simulink model "copia"  (R2019a)
settings: Solver=VariableStepAuto  StartTime=0.0  StopTime=1005  RelTol=1e-3
values from neighbouring files (symbols this model uses):
  alfa_cu = 3.9 * 10^(-3)    (= 0.0039)    [Datos.m]
  ba = 0.0113    [Calculo.m]
  beq = (bm+bl/r^2)    [Calculo.m]    (also in Untitled4.m; funciontrans.m)
  bm = 1.5 * 10^(-5)    (= 1.5e-05)    [Datos.m]
  Cts = 0.818    [Datos.m]
  Id0 = 0.5    [Datos.m]    (also in punto6plot.m)
  Jeq = (Jm+Jl/r^2)    [Calculo.m]    (also in Untitled4.m)
  Jeq1 = (Jm+Jlv(i)/r^2)    [Calculo.m]    (also in funciontrans.m)
  Koth = 6400    [Calculo.m]
  Kow = 3200^2    (= 10240000)    [Calculo.m]
  ksa = 9.04    [Calculo.m]
  ksia = 2892.8    [Calculo.m]
  lambda_m_r = 0.01546    [Datos.m]
  Ld = 6.6e-3    (= 0.0066)    [Datos.m]
  Lls = 0.8e-3    (= 0.0008)    [Datos.m]
  Lq = 5.8e-3    (= 0.0058)    [Datos.m]
  Pp = 3    [Datos.m]
  r = 314.3008    [Datos.m]
  Rts_amb = 146.7    [Datos.m]
undefined symbols (not defined in the file or in its folder): KowI, KT, KTd, magnitude, R0, Rd, Rq, sigbuilder_block, Tau, W0, W1
settings Model: Creator=renzo  LastModifiedBy=renzo

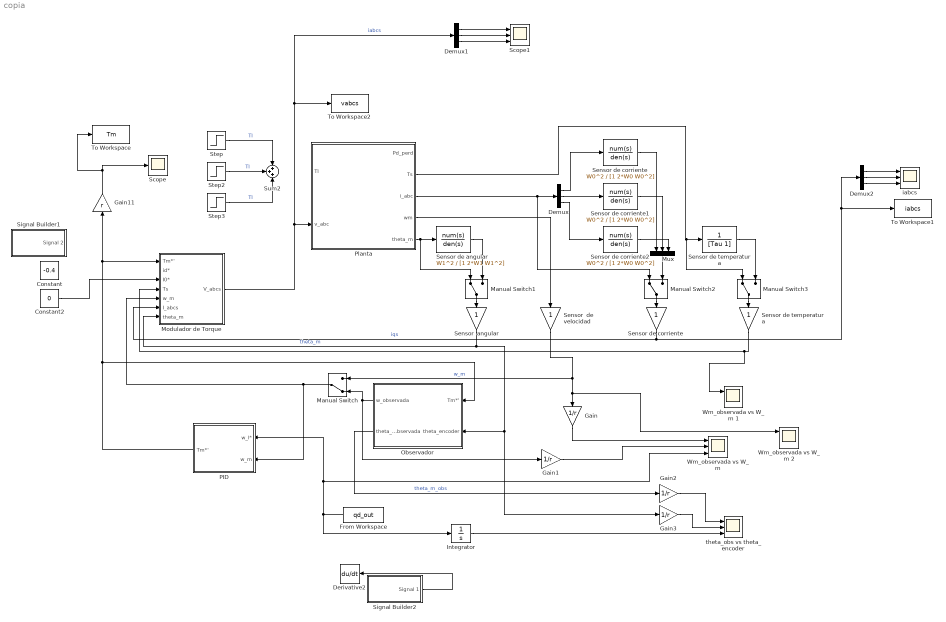
== system copia ==
  Constant : Constant  Value=-0.4
  Constant2 : Constant  Value=0
  Demux : Demux  Outputs=3
  Demux1 : Demux  Outputs=3
  Demux2 : Demux  Outputs=3
  Derivative2 : Derivative
  From Workspace : FromWorkspace  VariableName=qd_out  SampleTime=0
  Gain{,1..3} (4 alike) : Gain  Gain=1/r
  Gain11 : Gain  Gain=r
  Integrator : Integrator
  Manual Switch : ManualSwitch  CurrentSetting=0
  Manual Switch1 : ManualSwitch
  Manual Switch2 : ManualSwitch
  Manual Switch3 : ManualSwitch
  Modulador de Torque : Subsystem
  Mux : Mux  Inputs=3
  Observador : Subsystem
  PID : Subsystem
  Planta : Subsystem
  Scope : Scope
  Scope1 : Scope  NumInputPorts=3
  Sensor  angular : Gain
  Sensor  de velocidad : Gain
  Sensor de angular : TransferFcn  Numerator=W1^2  Denominator=[1 2*W1 W1^2]
  Sensor de corriente : TransferFcn  Numerator=W0^2  Denominator=[1 2*W0 W0^2]
  "Sensor de corriente " : Gain
  Sensor de corriente1 : TransferFcn  Numerator=W0^2  Denominator=[1 2*W0 W0^2]
  Sensor de corriente2 : TransferFcn  Numerator=W0^2  Denominator=[1 2*W0 W0^2]
  Sensor de temperatura : TransferFcn  Numerator=1  Denominator=[Tau 1]
  "Sensor de temperatura " : Gain
  Signal Builder1 : Subsystem  Tag=STV Subsys  LoadFcn=sigbuilder_block('load');  StartFcn=sigbuilder_block('start');  StopFcn=sigbuilder_block('stop');  ClipboardFcn=sigbuilder_block('clipboard');  mask(Sigbuilder block){tuvar=[0:10]}
      mask help: Simulink:masks:SigbuilderBlock_MD
      mask init:
      | if ~strcmp(get_param(bdroot(gcbh),'SimulationStatus'),'stopped') tuvar = sigbuilder_block('maskInit'); end
      settings: CopyFcn=sigbuilder_block('copy');  DeleteFcn=sigbuilder_block('delete');  ModelCloseFcn=sigbuilder_block('modelClose');  PreSaveFcn=sigbuilder_block('preSave');  PauseFcn=sigbuilder_block('pause');  ContinueFcn=sigbuilder_block('continue');  NameChangeFcn=sigbuilder_block('namechange');  OpenFcn=sigbuilder_block('open',[6 126.75 550.5 359.25 ]);  CloseFcn=sigbuilder_block('close');
      mask Display: plot(0, 0, 100, 100,[2, 2, 32, 32, 2], [68, 8, 8, 68, 68],[32, 2], [38, 38], [32, 19, 2],[53, 60, 44], [32, 17, 17, 2],[16, 16, 31, 31]);txt = getActiveGroup(gcbh);text(2, 100, txt,'verticalAlignment', 'top');
  Signal Builder2 : Subsystem  Tag=STV Subsys  LoadFcn=sigbuilder_block('load');  StartFcn=sigbuilder_block('start');  StopFcn=sigbuilder_block('stop');  ClipboardFcn=sigbuilder_block('clipboard');  mask(Sigbuilder block){tuvar=[0:10]}
      mask help: Simulink:masks:SigbuilderBlock_MD
      mask init:
      | if ~strcmp(get_param(bdroot(gcbh),'SimulationStatus'),'stopped') tuvar = sigbuilder_block('maskInit'); end
      settings: CopyFcn=sigbuilder_block('copy');  DeleteFcn=sigbuilder_block('delete');  ModelCloseFcn=sigbuilder_block('modelClose');  PreSaveFcn=sigbuilder_block('preSave');  PauseFcn=sigbuilder_block('pause');  ContinueFcn=sigbuilder_block('continue');  NameChangeFcn=sigbuilder_block('namechange');  OpenFcn=sigbuilder_block('open',[437.6 153 550.4 359.25 ]);  CloseFcn=sigbuilder_block('close');
      mask Display: plot(0, 0, 100, 100,[2, 2, 32, 32, 2], [68, 8, 8, 68, 68],[32, 2], [38, 38], [32, 19, 2],[53, 60, 44], [32, 17, 17, 2],[16, 16, 31, 31]);txt = getActiveGroup(gcbh);text(2, 100, txt,'verticalAlignment', 'top');
  Step : Step  Time=0.3  After=6.28  SampleTime=0
  Step2 : Step  Time=0.5  After=-2*6.28  SampleTime=0
  Step3 : Step  Time=0.9  After=6.28  SampleTime=0
  Sum2 : Sum  Inputs=+++
  To Workspace : ToWorkspace  VariableName=Tm  SaveFormat=Timeseries  SampleTime=-1
  To Workspace1 : ToWorkspace  VariableName=iabcs  SaveFormat=Timeseries  SampleTime=-1
  To Workspace2 : ToWorkspace  VariableName=vabcs  SaveFormat=Timeseries  SampleTime=-1
  "Wm_observada vs W_m " : Scope  NumInputPorts=3
  Wm_observada vs W_m 1 : Scope  NumInputPorts=3
  Wm_observada vs W_m 2 : Scope  NumInputPorts=3
  iabcs : Scope  NumInputPorts=3
  theta_obs vs theta_encoder : Scope  NumInputPorts=3
  wires:
  Planta/3(i_abc) -> Manual Switch2/1, Demux/1
  Planta/4(wm) -> Sensor  de velocidad/1
  Sensor  angular/1 -> Observador/2(theta_encoder), Gain3/1, Modulador de Torque/7(theta_m)  "theta_m"
  Manual Switch/1 -> PID/2(w_m), Modulador de Torque/5("w_m ")
  "Sensor de corriente "/1 -> To Workspace1/1, Demux2/1, Modulador de Torque/6(I_abcs)  "iqs"
  "Sensor de temperatura "/1 -> Wm_observada vs W_m 1/1, Modulador de Torque/4(Ts)
  Gain/1 -> "Wm_observada vs W_m "/1
  Observador/2(theta_observada) -> Gain2/1  "theta_m_obs"
  Gain1/1 -> "Wm_observada vs W_m "/2
  Gain2/1 -> theta_obs vs theta_encoder/1
  Gain3/1 -> theta_obs vs theta_encoder/2
  Sensor  de velocidad/1 -> Manual Switch/1, Wm_observada vs W_m 2/1, Gain/1  "w_m"
  Observador/1(w_observada) -> Gain1/1, Manual Switch/2
  Step2/1 -> Sum2/2  "Tl"
  Step/1 -> Sum2/1  "Tl"
  Step3/1 -> Sum2/3  "Tl"
  Constant2/1 -> Modulador de Torque/3(I0*)
  PID/1(Tm*') -> Observador/1(Tm*'), Gain11/1, Modulador de Torque/1(Tm*')
  Demux/1 -> Sensor de corriente/1
  Demux/2 -> Sensor de corriente1/1
  Demux/3 -> Sensor de corriente2/1
  Mux/1 -> Manual Switch2/2
  Sensor de corriente/1 -> Mux/1
  Sensor de corriente1/1 -> Mux/2
  Sensor de corriente2/1 -> Mux/3
  Planta/2(Ts) -> Manual Switch3/1, Sensor de temperatura/1
  Planta/5(theta_m) -> Sensor de angular/1, Manual Switch1/1
  Sensor de angular/1 -> Manual Switch1/2
  Integrator/1 -> theta_obs vs theta_encoder/3
  Manual Switch1/1 -> Sensor  angular/1
  Manual Switch3/1 -> "Sensor de temperatura "/1
  Sensor de temperatura/1 -> Manual Switch3/2
  Manual Switch2/1 -> "Sensor de corriente "/1
  Gain11/1 -> To Workspace/1, Scope/1
  Signal Builder2/1(Signal 1) -> Derivative2/1
  Modulador de Torque/1(V_abcs) -> Demux1/1, To Workspace2/1, Planta/2(v_abc)  "iabcs"
  Demux1/2 -> Scope1/2
  Demux1/1 -> Scope1/1
  Demux1/3 -> Scope1/3
  Demux2/1 -> iabcs/1
  Demux2/2 -> iabcs/2
  Demux2/3 -> iabcs/3
  From Workspace/1 -> Integrator/1, "Wm_observada vs W_m "/3, PID/1(w_l*)

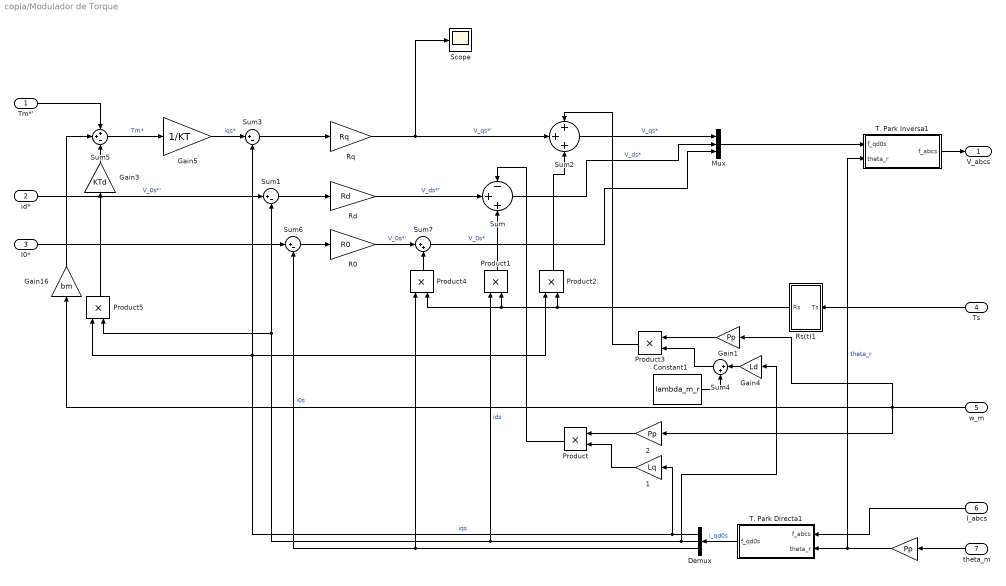
== system copia/Modulador de Torque ==
  Tm*' : Inport
  id* : Inport  Port=2
  I0* : Inport  Port=3
  Ts : Inport  Port=4
  "w_m " : Inport  Port=5
  I_abcs : Inport  Port=6
  theta_m : Inport  Port=7
  " " : Gain  Gain=Pp
  " 1" : Gain  Gain=Lq
  " 2" : Gain  Gain=Pp
  Constant1 : Constant  Value=lambda_m_r
  Demux : Demux  Outputs=3
  Gain1 : Gain  Gain=Pp
  Gain16 : Gain  Gain=bm
  Gain3 : Gain  Gain=KTd
  Gain4 : Gain  Gain=Ld
  Gain5 : Gain  Gain=1/KT
  Mux : Mux  Inputs=3
  Product{,1..5} (6 alike) : Product
  R0 : Gain  Gain=R0
  Rd : Gain  Gain=Rd
  Rq : Gain  Gain=Rq
  Rs(t)1 : Subsystem
  Scope : Scope
  Sum : Sum  Inputs=-++
  Sum1 : Sum  Inputs=|+-
  Sum2 : Sum  Inputs=+++
  Sum3 : Sum  Inputs=|+-
  Sum4 : Sum  Inputs=|++
  Sum5 : Sum  Inputs=++-
  Sum6 : Sum  Inputs=|+-
  Sum7 : Sum  Inputs=|++
  T. Park Directa1 : Subsystem
  T. Park Inversa1 : Subsystem
  V_abcs : Outport
  wires:
  theta_m/1 -> " "/1
  Product3/1 -> Sum2/1
  Rs(t)1/1(Rs) -> Product2/2, Product1/2, Product4/2
  Sum/1 -> Mux/2  "V_ds*"
  Product1/1 -> Sum/3
  Sum1/1 -> Rd/1
  Demux/3 -> Sum6/2, Product4/1  "i0s"
  Rd/1 -> Sum/2  "V_ds*'"
  Gain16/1 -> Sum5/2
  Sum2/1 -> Mux/1  "V_qs*"
  Gain4/1 -> Sum4/1
  Sum6/1 -> R0/1
  Sum4/1 -> Product3/2
  Product2/1 -> Sum2/3
  " "/1 -> T. Park Directa1/2(theta_r), T. Park Inversa1/2(theta_r)  "theta_r"
  Sum7/1 -> Mux/3  "V_0s*"
  Mux/1 -> T. Park Inversa1/1(f_qd0s)
  T. Park Directa1/1(f_qd0s) -> Demux/1  "i_qd0s"
  Product/1 -> Sum/1
  Tm*'/1 -> Sum5/1
  Sum5/1 -> Gain5/1  "Tm*"
  " 1"/1 -> Product/2
  Demux/1 -> " 1"/1, Product2/1, Product5/1, Sum3/2  "iqs"
  Sum3/1 -> Rq/1
  I0*/1 -> Sum6/1
  Demux/2 -> Gain4/1, Product5/2, Sum1/2, Product1/1  "ids"
  Rq/1 -> Scope/1, Sum2/2  "V_qs*'"
  Constant1/1 -> Sum4/2
  T. Park Inversa1/1(f_abcs) -> V_abcs/1
  R0/1 -> Sum7/1  "V_0s*'"
  " 2"/1 -> Product/1
  I_abcs/1 -> T. Park Directa1/1(f_abcs)
  Product4/1 -> Sum7/2
  Gain1/1 -> Product3/1
  Ts/1 -> Rs(t)1/1(Ts)
  "w_m "/1 -> " 2"/1, Gain16/1, Gain1/1
  Gain5/1 -> Sum3/1  "iqs*"
  Product5/1 -> Gain3/1
  Gain3/1 -> Sum5/3
  id*/1 -> Sum1/1  "V_0s*'"

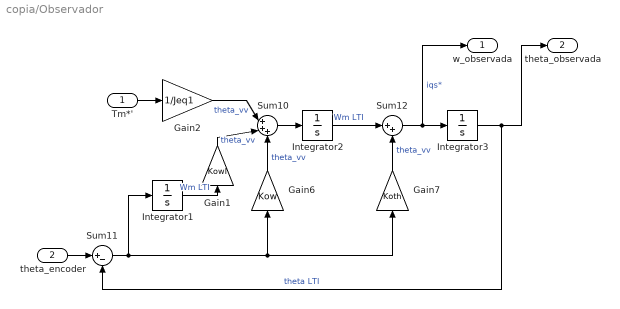
== system copia/Observador ==
  Tm*' : Inport
  theta_encoder : Inport  Port=2
  Gain1 : Gain  Gain=KowI
  Gain2 : Gain  Gain=1/Jeq1
  Gain6 : Gain  Gain=Kow
  Gain7 : Gain  Gain=Koth
  Integrator1 : Integrator
  Integrator2 : Integrator
  Integrator3 : Integrator
  Sum10 : Sum  Inputs=|+++
  Sum11 : Sum  Inputs=|+-
  Sum12 : Sum  Inputs=|++
  w_observada : Outport
  theta_observada : Outport  Port=2
  wires:
  Gain6/1 -> Sum10/3  "theta_vv"
  Sum10/1 -> Integrator2/1
  Gain2/1 -> Sum10/1  "theta_vv"
  Integrator2/1 -> Sum12/1  "Wm LTI"
  Gain7/1 -> Sum12/2  "theta_vv"
  Sum12/1 -> w_observada/1, Integrator3/1  "iqs*"
  Integrator3/1 -> theta_observada/1, Sum11/2  "theta LTI"
  Tm*'/1 -> Gain2/1
  theta_encoder/1 -> Sum11/1
  Sum11/1 -> Integrator1/1, Gain7/1, Gain6/1
  Integrator1/1 -> Gain1/1  "Wm LTI"
  Gain1/1 -> Sum10/2  "theta_vv"

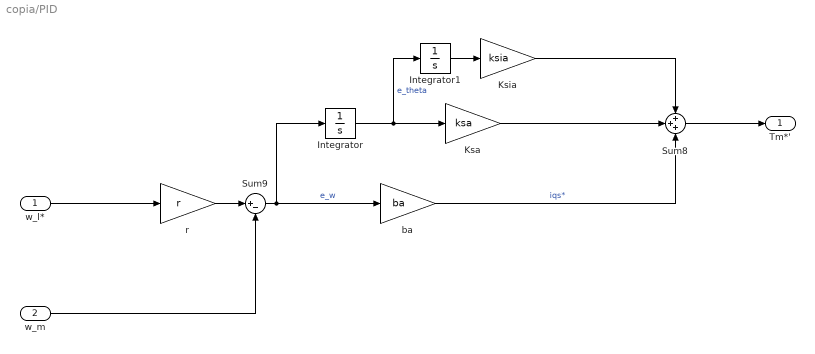
== system copia/PID ==
  w_l* : Inport
  w_m : Inport  Port=2
  Integrator : Integrator
  Integrator1 : Integrator
  Ksa : Gain  Gain=ksa
  Ksia : Gain  Gain=ksia
  Sum8 : Sum  Inputs=+++
  Sum9 : Sum  Inputs=|+-
  ba : Gain  Gain=ba
  r : Gain  Gain=r
  Tm*' : Outport
  wires:
  Integrator/1 -> Integrator1/1, Ksa/1  "e_theta"
  Sum9/1 -> Integrator/1, ba/1  "e_w"
  Ksa/1 -> Sum8/2
  ba/1 -> Sum8/3  "iqs*"
  Ksia/1 -> Sum8/1
  r/1 -> Sum9/1
  w_m/1 -> Sum9/2
  Integrator1/1 -> Ksia/1
  w_l*/1 -> r/1
  Sum8/1 -> Tm*'/1

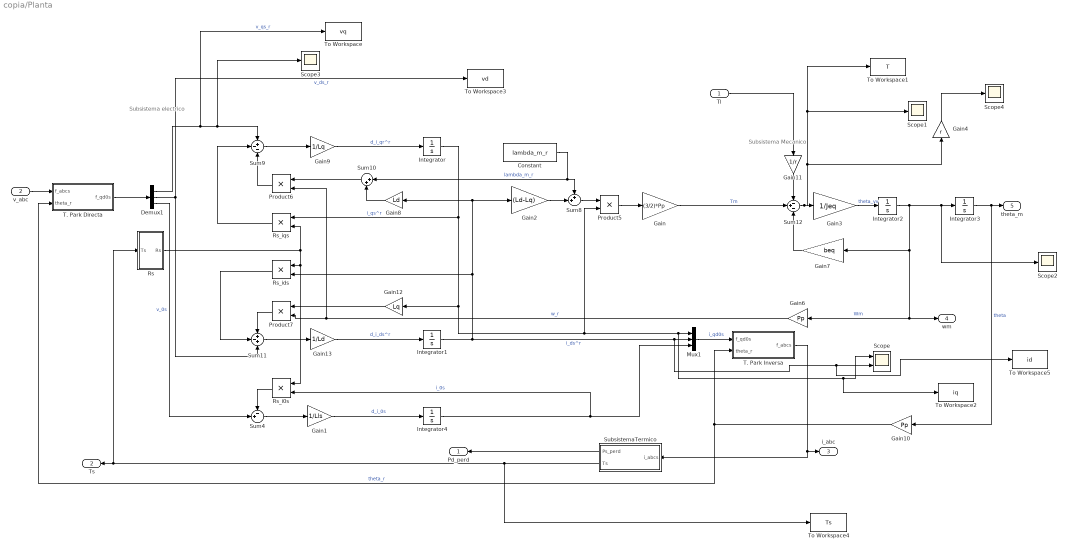
== system copia/Planta ==
  note: Subsistema Mecanico
  note: Subsistema electrico
  Tl : Inport
  v_abc : Inport  Port=2
  Constant : Constant  Value=lambda_m_r
  Demux1 : Demux  Outputs=3
  Gain : Gain  Gain=(3/2)*Pp
  Gain1 : Gain  Gain=1/Lls
  Gain10 : Gain  Gain=Pp
  Gain11 : Gain  Gain=1/r
  Gain12 : Gain  Gain=Lq
  Gain13 : Gain  Gain=1/Ld
  Gain2 : Gain  Gain=(Ld-Lq)
  Gain3 : Gain  Gain=1/Jeq
  Gain4 : Gain  Gain=r
  Gain6 : Gain  Gain=Pp
  Gain7 : Gain  Gain=beq
  Gain8 : Gain  Gain=Ld
  Gain9 : Gain  Gain=1/Lq
  Integrator{,2..4} (4 alike) : Integrator
  Integrator1 : Integrator  InitialCondition=Id0
  Mux1 : Mux  Inputs=3
  Product5 : Product
  Product6 : Product
  Product7 : Product
  Rs : Subsystem
  Rs_i0s : Product
  Rs_ids : Product
  Rs_iqs : Product
  Scope : Scope  NumInputPorts=2
  Scope{1..4} (4 alike) : Scope
  SubsistemaTermico : Subsystem
  Sum10 : Sum  Inputs=|++
  Sum11 : Sum  Inputs=+-+
  Sum12 : Sum  Inputs=-+-
  Sum4 : Sum  Inputs=-+|
  Sum8 : Sum  Inputs=++|
  Sum9 : Sum  Inputs=+--
  T. Park Directa : Subsystem
  T. Park Inversa : Subsystem
  To Workspace : ToWorkspace  VariableName=vq  SaveFormat=Timeseries  SampleTime=-1
  To Workspace1 : ToWorkspace  VariableName=T  SaveFormat=Timeseries  SampleTime=-1
  To Workspace2 : ToWorkspace  VariableName=iq  SaveFormat=Timeseries  SampleTime=-1
  To Workspace3 : ToWorkspace  VariableName=vd  SaveFormat=Timeseries  SampleTime=-1
  To Workspace4 : ToWorkspace  VariableName=Ts  SaveFormat=Timeseries  SampleTime=-1
  To Workspace5 : ToWorkspace  VariableName=id  SaveFormat=Timeseries  SampleTime=-1
  Pd_perd : Outport
  Ts : Outport  Port=2
  i_abc : Outport  Port=3
  wm : Outport  Port=4
  theta_m : Outport  Port=5
  wires:
  T. Park Inversa/1(f_abcs) -> SubsistemaTermico/1(i_abcs), i_abc/1
  SubsistemaTermico/1(Ps_perd) -> Pd_perd/1
  Gain10/1 -> T. Park Directa/2(theta_r), T. Park Inversa/2(theta_r)  "theta_r"
  Mux1/1 -> T. Park Inversa/1(f_qd0s)  "i_qd0s"
  v_abc/1 -> T. Park Directa/1(f_abcs)
  Gain6/1 -> Product6/2, Product7/2  "w_r"
  Sum8/1 -> Product5/1
  T. Park Directa/1(f_qd0s) -> Demux1/1
  Gain9/1 -> Integrator/1  "d_i_qr^r"
  Gain12/1 -> Product7/1
  Demux1/2 -> Sum11/3, To Workspace3/1  "v_ds_r"
  Rs_i0s/1 -> Sum4/1
  Rs_ids/1 -> Sum11/2
  Demux1/3 -> Sum4/2  "v_0s"
  Gain8/1 -> Sum10/2
  Sum4/1 -> Gain1/1
  Sum10/1 -> Product6/1
  Gain2/1 -> Sum8/2
  Product7/1 -> Sum11/1
  Rs_iqs/1 -> Sum9/2
  Sum11/1 -> Gain13/1
  SubsistemaTermico/2(Ts) -> To Workspace4/1, Rs/1(Ts), Ts/1
  Gain1/1 -> Integrator4/1  "d_i_0s"
  Integrator4/1 -> Mux1/3, Rs_i0s/2  "i_0s"
  Rs/1(Rs) -> Rs_i0s/1, Rs_ids/1, Rs_iqs/2
  Sum9/1 -> Gain9/1
  Integrator1/1 -> To Workspace5/1, Scope/2, Mux1/2, Rs_ids/2, Gain2/1, Gain8/1  "i_ds^r"
  Product6/1 -> Sum9/3
  Integrator/1 -> Gain12/1, To Workspace2/1, Scope/1, Mux1/1, Product5/2, Rs_iqs/1  "i_qs^r"
  Constant/1 -> Sum8/1, Sum10/1  "lambda_m_r"
  Demux1/1 -> To Workspace/1, Scope3/1, Sum9/1  "v_qs_r"
  Gain13/1 -> Integrator1/1  "d_i_ds^r"
  Tl/1 -> Gain11/1
  Integrator3/1 -> Gain10/1, theta_m/1  "theta"
  Gain11/1 -> Sum12/1
  Integrator2/1 -> Scope2/1, Integrator3/1, Gain7/1, Gain6/1, wm/1  "Wm"
  Product5/1 -> Gain/1
  Gain/1 -> Sum12/2  "Tm"
  Gain3/1 -> Integrator2/1  "theta_vv"
  Gain7/1 -> Sum12/3
  Sum12/1 -> Gain4/1, Scope1/1, To Workspace1/1, Gain3/1
  Gain4/1 -> Scope4/1

== system copia/Signal Builder1 ==
  Demux : Demux  Tag=STV Demux  Outputs=1
  FromWs : FromWorkspace  Tag=STV FromWs  VariableName=tuvar  SampleTime=0
      SigBuilderData=|
      | common.afterFinalStr = 'Extrapolate'
      | common.sampleTime = 0
      | dataSet.timeRange = [0 10]
      | dataSet.name = 'Group 1'
      | sbobj.Groups.Name = 'Group 1'
      | sbobj.Groups.Signals.Name = 'Signal 2'
      | sbobj.Groups.Signals.XData = [0 0.1 0.1 0.7 0.7 10]
      | sbobj.Groups.Signals.YData = [0 0 0.0063 0.0063 0 0]
  Signal 2 : Outport  Tag=STV Outport
  wires:
  FromWs/1 -> Demux/1
  Demux/1 -> Signal 2/1

== system copia/Signal Builder2 ==
  Demux : Demux  Tag=STV Demux  Outputs=1
  FromWs : FromWorkspace  Tag=STV FromWs  VariableName=tuvar  SampleTime=0
      SigBuilderData=|
      | common.afterFinalStr = 'Extrapolate'
      | common.sampleTime = 0
      | dataSet.timeRange = [0 20]
      | dataSet.name = 'Group 1'
      | sbobj.Groups.Name = 'Group 1'
      | sbobj.Groups.Signals.Name = 'Signal 1'
      | sbobj.Groups.Signals.XData = [0 1 6 11 16 20]
      | sbobj.Groups.Signals.YData = [0 0 6.28318530718 6.28318530718 0 0]
      | sbobj.Groups.TimeRange = [0 20]
  Signal 1 : Outport  Tag=STV Outport
  wires:
  Demux/1 -> Signal 1/1
  FromWs/1 -> Demux/1

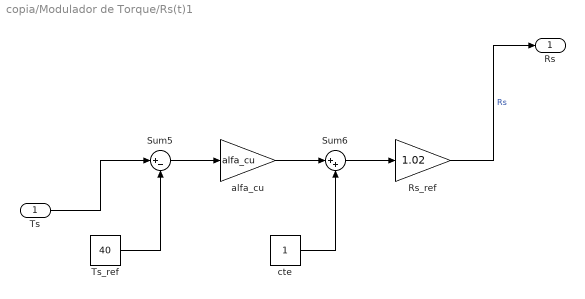
== system copia/Modulador de Torque/Rs(t)1 ==
  Ts : Inport
  Rs_ref : Gain  Gain=1.02
  Sum5 : Sum  Inputs=|+-
  Sum6 : Sum  Inputs=|++
  Ts_ref : Constant  Value=40
  alfa_cu : Gain  Gain=alfa_cu
  cte : Constant
  Rs : Outport
  wires:
  alfa_cu/1 -> Sum6/1
  Sum6/1 -> Rs_ref/1
  Rs_ref/1 -> Rs/1  "Rs"
  Ts_ref/1 -> Sum5/2
  cte/1 -> Sum6/2
  Ts/1 -> Sum5/1
  Sum5/1 -> alfa_cu/1

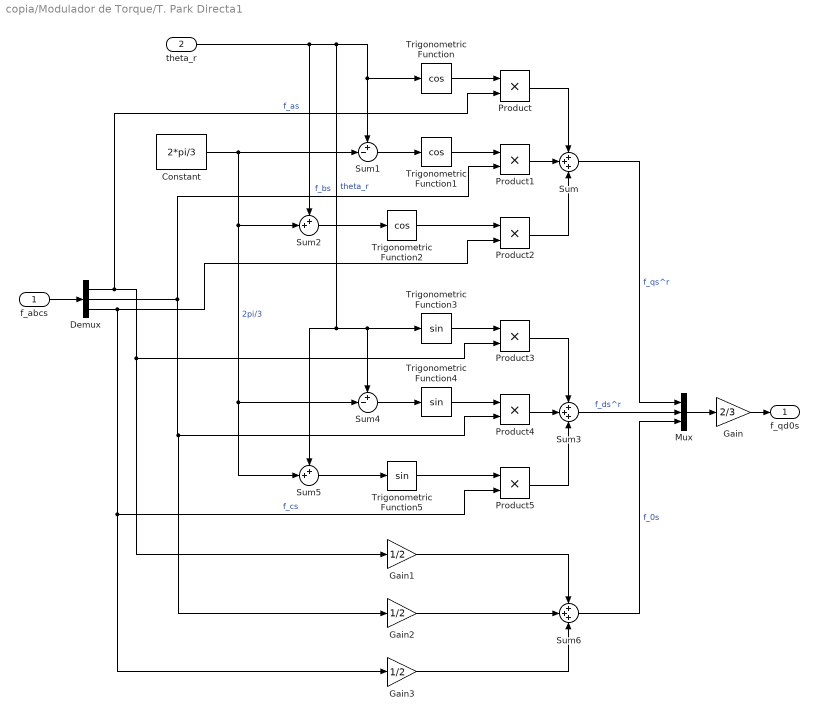
== system copia/Modulador de Torque/T. Park Directa1 ==
  f_abcs : Inport
  theta_r : Inport  Port=2
  Constant : Constant  Value=2*pi/3
  Demux : Demux  Outputs=3
  Gain : Gain  Gain=2/3
  Gain1 : Gain  Gain=1/2
  Gain2 : Gain  Gain=1/2
  Gain3 : Gain  Gain=1/2
  Mux : Mux  Inputs=3
  Product{,1..5} (6 alike) : Product
  Sum : Sum  Inputs=3
  Sum1 : Sum  Inputs=+-|
  Sum2 : Sum  Inputs=++|
  Sum3 : Sum  Inputs=3
  Sum4 : Sum  Inputs=+-|
  Sum5 : Sum  Inputs=++|
  Sum6 : Sum  Inputs=3
  Trigonometric Function : Trigonometry  Operator=cos
  Trigonometric Function1 : Trigonometry  Operator=cos
  Trigonometric Function2 : Trigonometry  Operator=cos
  Trigonometric Function3 : Trigonometry
  Trigonometric Function4 : Trigonometry
  Trigonometric Function5 : Trigonometry
  f_qd0s : Outport  VectorParamsAs1DForOutWhenUnconnected=on
  wires:
  Mux/1 -> Gain/1
  f_abcs/1 -> Demux/1
  Demux/1 -> Gain1/1, Product3/2, Product/2  "f_as"
  Demux/2 -> Gain2/1, Product4/2, Product1/2  "f_bs"
  Demux/3 -> Gain3/1, Product5/2, Product2/2  "f_cs"
  Sum/1 -> Mux/1  "f_qs^r"
  Gain/1 -> f_qd0s/1
  Trigonometric Function/1 -> Product/1
  Product/1 -> Sum/1
  Sum1/1 -> Trigonometric Function1/1
  Constant/1 -> Sum5/2, Sum4/2, Sum2/2, Sum1/2  "2pi/3"
  Trigonometric Function1/1 -> Product1/1
  Product1/1 -> Sum/2
  Product2/1 -> Sum/3
  Trigonometric Function2/1 -> Product2/1
  Sum2/1 -> Trigonometric Function2/1
  Product4/1 -> Sum3/2
  Trigonometric Function5/1 -> Product5/1
  Sum5/1 -> Trigonometric Function5/1
  Product5/1 -> Sum3/3
  Product3/1 -> Sum3/1
  Trigonometric Function4/1 -> Product4/1
  Sum4/1 -> Trigonometric Function4/1
  Sum3/1 -> Mux/2  "f_ds^r"
  Trigonometric Function3/1 -> Product3/1
  theta_r/1 -> Sum5/1, Sum4/1, Trigonometric Function3/1, Trigonometric Function/1, Sum1/1, Sum2/1  "theta_r"
  Sum6/1 -> Mux/3  "f_0s"
  Gain3/1 -> Sum6/3
  Gain1/1 -> Sum6/1
  Gain2/1 -> Sum6/2

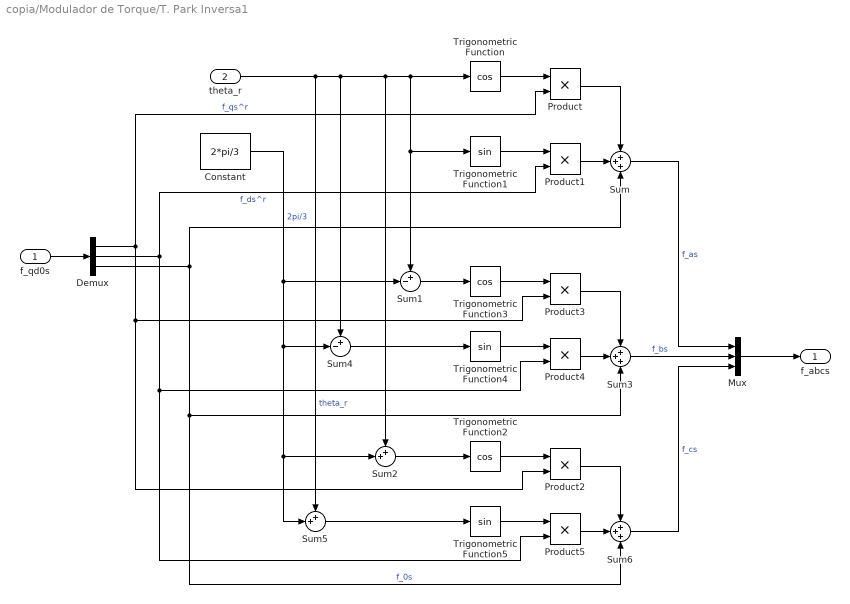
== system copia/Modulador de Torque/T. Park Inversa1 ==
  f_qd0s : Inport
  theta_r : Inport  Port=2
  Constant : Constant  Value=2*pi/3
  Demux : Demux  Outputs=3
  Mux : Mux  Inputs=3
  Product{,1..5} (6 alike) : Product
  Sum : Sum  Inputs=3
  Sum1 : Sum  Inputs=+-|
  Sum2 : Sum  Inputs=++|
  Sum3 : Sum  Inputs=3
  Sum4 : Sum  Inputs=+-|
  Sum5 : Sum  Inputs=++|
  Sum6 : Sum  Inputs=3
  Trigonometric Function : Trigonometry  Operator=cos
  Trigonometric Function1 : Trigonometry
  Trigonometric Function2 : Trigonometry  Operator=cos
  Trigonometric Function3 : Trigonometry  Operator=cos
  Trigonometric Function4 : Trigonometry
  Trigonometric Function5 : Trigonometry
  f_abcs : Outport  VectorParamsAs1DForOutWhenUnconnected=on
  wires:
  Trigonometric Function4/1 -> Product4/1
  f_qd0s/1 -> Demux/1
  Trigonometric Function/1 -> Product/1
  Constant/1 -> Sum1/2, Sum4/2, Sum2/2, Sum5/2  "2pi/3"
  Product1/1 -> Sum/2
  Mux/1 -> f_abcs/1
  Sum6/1 -> Mux/3  "f_cs"
  Product/1 -> Sum/1
  theta_r/1 -> Trigonometric Function/1, Trigonometric Function1/1, Sum1/1, Sum2/1, Sum4/1, Sum5/1  "theta_r"
  Product4/1 -> Sum3/2
  Sum3/1 -> Mux/2  "f_bs"
  Trigonometric Function1/1 -> Product1/1
  Sum/1 -> Mux/1  "f_as"
  Trigonometric Function3/1 -> Product3/1
  Product3/1 -> Sum3/1
  Sum4/1 -> Trigonometric Function4/1
  Demux/1 -> Product2/2, Product3/2, Product/2  "f_qs^r"
  Demux/2 -> Product5/2, Product4/2, Product1/2  "f_ds^r"
  Demux/3 -> Sum/3, Sum6/3, Sum3/3  "f_0s"
  Sum1/1 -> Trigonometric Function3/1
  Sum5/1 -> Trigonometric Function5/1
  Trigonometric Function5/1 -> Product5/1
  Trigonometric Function2/1 -> Product2/1
  Product2/1 -> Sum6/1
  Product5/1 -> Sum6/2
  Sum2/1 -> Trigonometric Function2/1

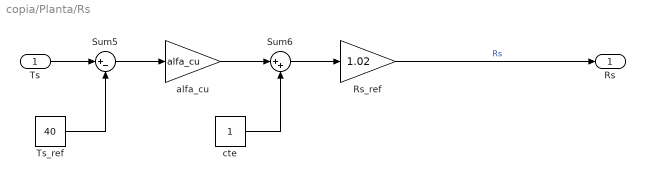
== system copia/Planta/Rs ==
  Ts : Inport
  Rs_ref : Gain  Gain=1.02
  Sum5 : Sum  Inputs=|+-
  Sum6 : Sum  Inputs=|++
  Ts_ref : Constant  Value=40
  alfa_cu : Gain  Gain=alfa_cu
  cte : Constant
  Rs : Outport
  wires:
  Ts_ref/1 -> Sum5/2
  Sum5/1 -> alfa_cu/1
  Sum6/1 -> Rs_ref/1
  Ts/1 -> Sum5/1
  alfa_cu/1 -> Sum6/1
  cte/1 -> Sum6/2
  Rs_ref/1 -> Rs/1  "Rs"

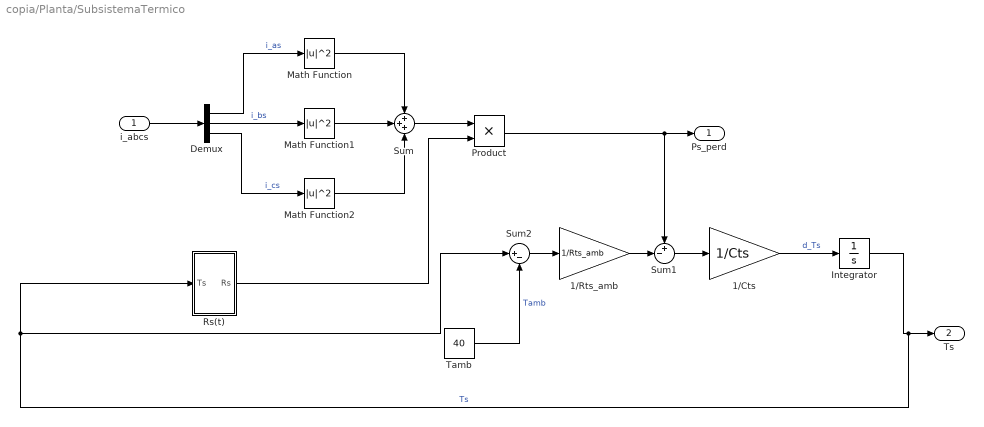
== system copia/Planta/SubsistemaTermico ==
  i_abcs : Inport
  1/Cts : Gain  Gain=1/Cts
  1/Rts_amb : Gain  Gain=1/Rts_amb
  Demux : Demux  Outputs=3
  Integrator : Integrator  InitialCondition=40
  Math Function : Math  Operator=magnitude^2  SaturateOnIntegerOverflow=on
  Math Function1 : Math  Operator=magnitude^2  SaturateOnIntegerOverflow=on
  Math Function2 : Math  Operator=magnitude^2  SaturateOnIntegerOverflow=on
  Product : Product
  Rs(t) : Subsystem
  Sum : Sum  Inputs=3
  Sum1 : Sum  Inputs=+-|
  Sum2 : Sum  Inputs=|+-
  Tamb : Constant  Value=40
  Ps_perd : Outport  VectorParamsAs1DForOutWhenUnconnected=on
  Ts : Outport  Port=2  VectorParamsAs1DForOutWhenUnconnected=on
  wires:
  i_abcs/1 -> Demux/1
  Demux/1 -> Math Function/1  "i_as"
  Demux/2 -> Math Function1/1  "i_bs"
  Demux/3 -> Math Function2/1  "i_cs"
  Math Function1/1 -> Sum/2
  Math Function/1 -> Sum/1
  Math Function2/1 -> Sum/3
  Sum/1 -> Product/1
  Product/1 -> Sum1/1, Ps_perd/1
  Tamb/1 -> Sum2/2  "Tamb"
  Sum2/1 -> 1/Rts_amb/1
  1/Rts_amb/1 -> Sum1/2
  Sum1/1 -> 1/Cts/1
  1/Cts/1 -> Integrator/1  "d_Ts"
  Integrator/1 -> Rs(t)/1(Ts), Sum2/1, Ts/1  "Ts"
  Rs(t)/1(Rs) -> Product/2

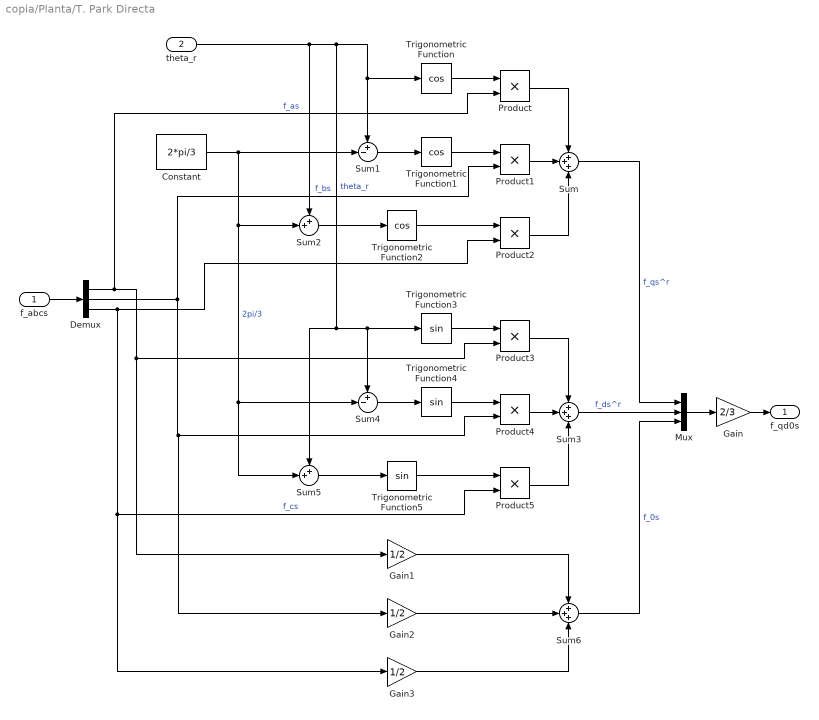
== system copia/Planta/T. Park Directa ==
  f_abcs : Inport
  theta_r : Inport  Port=2
  Constant : Constant  Value=2*pi/3
  Demux : Demux  Outputs=3
  Gain : Gain  Gain=2/3
  Gain1 : Gain  Gain=1/2
  Gain2 : Gain  Gain=1/2
  Gain3 : Gain  Gain=1/2
  Mux : Mux  Inputs=3
  Product{,1..5} (6 alike) : Product
  Sum : Sum  Inputs=3
  Sum1 : Sum  Inputs=+-|
  Sum2 : Sum  Inputs=++|
  Sum3 : Sum  Inputs=3
  Sum4 : Sum  Inputs=+-|
  Sum5 : Sum  Inputs=++|
  Sum6 : Sum  Inputs=3
  Trigonometric Function : Trigonometry  Operator=cos
  Trigonometric Function1 : Trigonometry  Operator=cos
  Trigonometric Function2 : Trigonometry  Operator=cos
  Trigonometric Function3 : Trigonometry
  Trigonometric Function4 : Trigonometry
  Trigonometric Function5 : Trigonometry
  f_qd0s : Outport  VectorParamsAs1DForOutWhenUnconnected=on
  wires:
  Mux/1 -> Gain/1
  f_abcs/1 -> Demux/1
  Demux/1 -> Gain1/1, Product3/2, Product/2  "f_as"
  Demux/2 -> Gain2/1, Product4/2, Product1/2  "f_bs"
  Demux/3 -> Gain3/1, Product5/2, Product2/2  "f_cs"
  Sum/1 -> Mux/1  "f_qs^r"
  Gain/1 -> f_qd0s/1
  Trigonometric Function/1 -> Product/1
  Product/1 -> Sum/1
  Sum1/1 -> Trigonometric Function1/1
  Constant/1 -> Sum5/2, Sum4/2, Sum2/2, Sum1/2  "2pi/3"
  Trigonometric Function1/1 -> Product1/1
  Product1/1 -> Sum/2
  Product2/1 -> Sum/3
  Trigonometric Function2/1 -> Product2/1
  Sum2/1 -> Trigonometric Function2/1
  Product4/1 -> Sum3/2
  Trigonometric Function5/1 -> Product5/1
  Sum5/1 -> Trigonometric Function5/1
  Product5/1 -> Sum3/3
  Product3/1 -> Sum3/1
  Trigonometric Function4/1 -> Product4/1
  Sum4/1 -> Trigonometric Function4/1
  Sum3/1 -> Mux/2  "f_ds^r"
  Trigonometric Function3/1 -> Product3/1
  theta_r/1 -> Sum5/1, Sum4/1, Trigonometric Function3/1, Trigonometric Function/1, Sum1/1, Sum2/1  "theta_r"
  Sum6/1 -> Mux/3  "f_0s"
  Gain3/1 -> Sum6/3
  Gain1/1 -> Sum6/1
  Gain2/1 -> Sum6/2

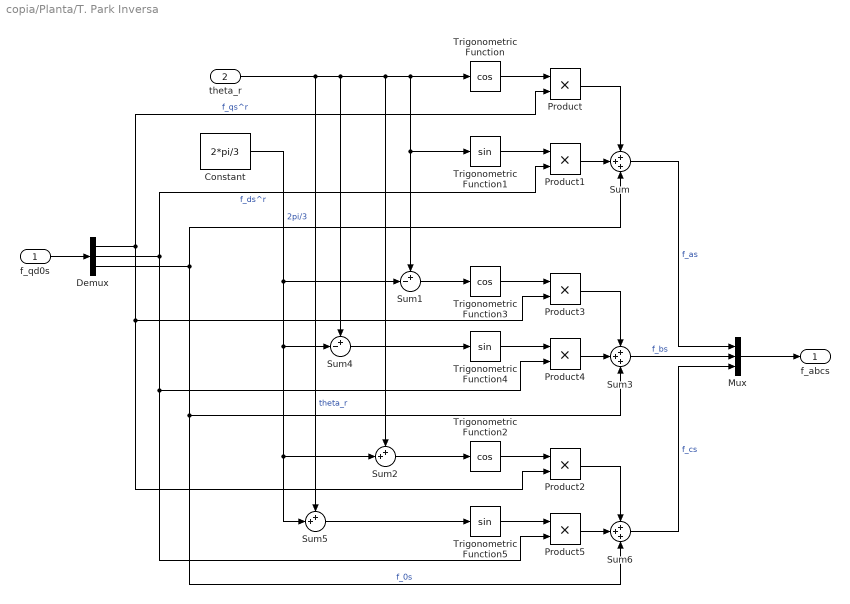
== system copia/Planta/T. Park Inversa ==
  f_qd0s : Inport
  theta_r : Inport  Port=2
  Constant : Constant  Value=2*pi/3
  Demux : Demux  Outputs=3
  Mux : Mux  Inputs=3
  Product{,1..5} (6 alike) : Product
  Sum : Sum  Inputs=3
  Sum1 : Sum  Inputs=+-|
  Sum2 : Sum  Inputs=++|
  Sum3 : Sum  Inputs=3
  Sum4 : Sum  Inputs=+-|
  Sum5 : Sum  Inputs=++|
  Sum6 : Sum  Inputs=3
  Trigonometric Function : Trigonometry  Operator=cos
  Trigonometric Function1 : Trigonometry
  Trigonometric Function2 : Trigonometry  Operator=cos
  Trigonometric Function3 : Trigonometry  Operator=cos
  Trigonometric Function4 : Trigonometry
  Trigonometric Function5 : Trigonometry
  f_abcs : Outport  VectorParamsAs1DForOutWhenUnconnected=on
  wires:
  Trigonometric Function4/1 -> Product4/1
  f_qd0s/1 -> Demux/1
  Trigonometric Function/1 -> Product/1
  Constant/1 -> Sum1/2, Sum4/2, Sum2/2, Sum5/2  "2pi/3"
  Product1/1 -> Sum/2
  Mux/1 -> f_abcs/1
  Sum6/1 -> Mux/3  "f_cs"
  Product/1 -> Sum/1
  theta_r/1 -> Trigonometric Function/1, Trigonometric Function1/1, Sum1/1, Sum2/1, Sum4/1, Sum5/1  "theta_r"
  Product4/1 -> Sum3/2
  Sum3/1 -> Mux/2  "f_bs"
  Trigonometric Function1/1 -> Product1/1
  Sum/1 -> Mux/1  "f_as"
  Trigonometric Function3/1 -> Product3/1
  Product3/1 -> Sum3/1
  Sum4/1 -> Trigonometric Function4/1
  Demux/1 -> Product2/2, Product3/2, Product/2  "f_qs^r"
  Demux/2 -> Product5/2, Product4/2, Product1/2  "f_ds^r"
  Demux/3 -> Sum/3, Sum6/3, Sum3/3  "f_0s"
  Sum1/1 -> Trigonometric Function3/1
  Sum5/1 -> Trigonometric Function5/1
  Trigonometric Function5/1 -> Product5/1
  Trigonometric Function2/1 -> Product2/1
  Product2/1 -> Sum6/1
  Product5/1 -> Sum6/2
  Sum2/1 -> Trigonometric Function2/1

== system copia/Planta/SubsistemaTermico/Rs(t) ==
  Ts : Inport
  Rs_ref : Gain  Gain=1.02
  Sum5 : Sum  Inputs=|+-
  Sum6 : Sum  Inputs=|++
  Ts_ref : Constant  Value=40
  alfa_cu : Gain  Gain=alfa_cu
  cte : Constant
  Rs : Outport
  wires:
  alfa_cu/1 -> Sum6/1
  Sum6/1 -> Rs_ref/1
  Rs_ref/1 -> Rs/1  "Rs"
  Ts_ref/1 -> Sum5/2
  cte/1 -> Sum6/2
  Ts/1 -> Sum5/1
  Sum5/1 -> alfa_cu/1
